simulink model "FIR_filter"  (R2020b)
settings: Solver=VariableStepAuto  StartTime=0.0  StopTime=10.0  RelTol=1e-3
settings Model: Creator=saadh  LastModifiedBy=saadh
settings DataIOCC: SaveOutput=off  SaveTime=off

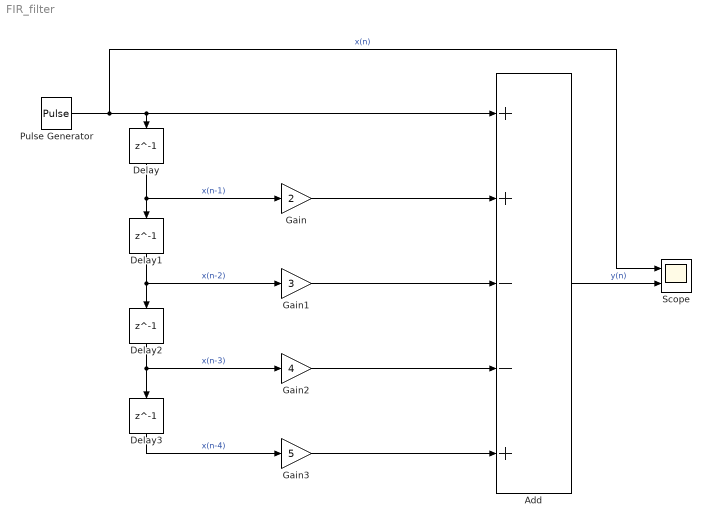
== system FIR_filter ==
  Add : Sum  Inputs=++--+
  Delay{,1..3} (4 alike) : Delay  DelayLength=1
  Gain : Gain  Gain=2
  Gain1 : Gain  Gain=3
  Gain2 : Gain  Gain=4
  Gain3 : Gain  Gain=5
  Pulse Generator : DiscretePulseGenerator  PulseType=Time based  Period=1  PulseWidth=5
  Scope : Scope  NumInputPorts=2
  wires:
  Gain2/1 -> Add/4
  Pulse Generator/1 -> Scope/1, Delay/1, Add/1  "x(n)"
  Gain1/1 -> Add/3
  Add/1 -> Scope/2  "y(n)"
  Delay1/1 -> Gain1/1, Delay2/1  "x(n-2)"
  Gain3/1 -> Add/5
  Delay/1 -> Gain/1, Delay1/1  "x(n-1)"
  Delay3/1 -> Gain3/1  "x(n-4)"
  Delay2/1 -> Gain2/1, Delay3/1  "x(n-3)"
  Gain/1 -> Add/2
